simulink model "messageEvents_example1"  (R2024b)
settings: Solver=VariableStepAuto  StartTime=0.0  StopTime=10.0  RelTol=1e-3
undefined symbols (not defined in the file): Call, Function
settings Model: Creator=optimus  LastModifiedBy=optimus

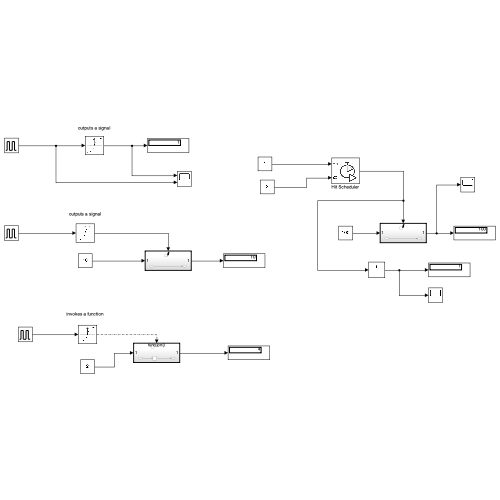
[thumbnail: Simulink's stored preview of the top-level diagram]
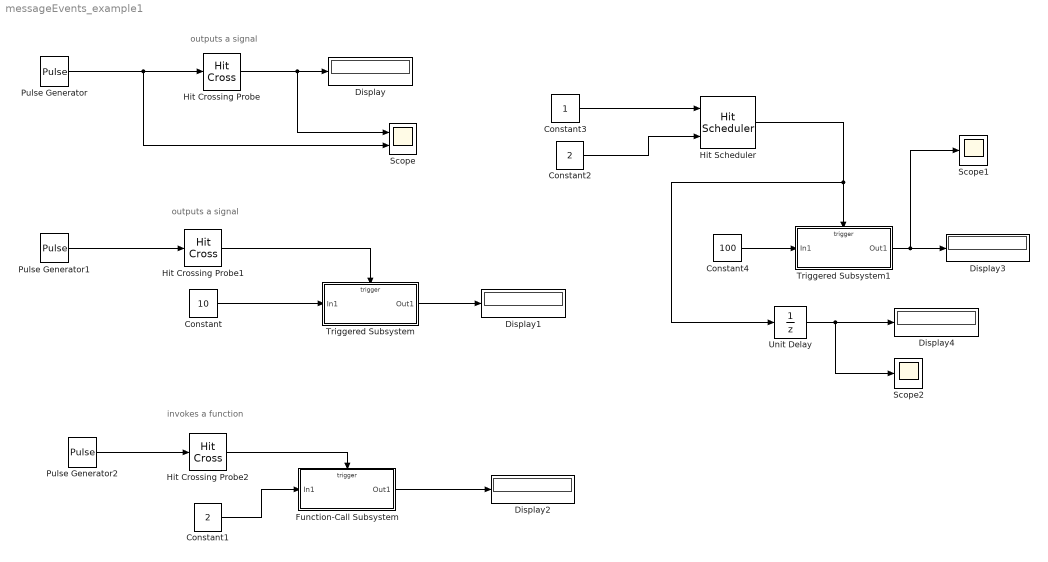
== system messageEvents_example1 ==
  note: invokes a function
  note: outputs a signal
  note: outputs a signal
  Constant : Constant  Value=10
  Constant1 : Constant  Value=2
  Constant2 : Constant  Value=2
  Constant3 : Constant  OutDataTypeStr=boolean
  Constant4 : Constant  Value=100
  Display{,1..4} (5 alike) : Display
  Function-Call Subsystem : Subsystem  TreatAsAtomicUnit=on
  Hit Crossing Probe : HitCross  HitCrossingDirection=rising
  Hit Crossing Probe1 : HitCross  HitCrossingDirection=rising
  Hit Crossing Probe2 : HitCross  HitCrossingDirection=rising  HitCrossingOutputType=Function-Call
  Hit Scheduler : HitScheduler
  Pulse Generator : DiscretePulseGenerator  PulseType=Time based  PulseWidth=50
  Pulse Generator1 : DiscretePulseGenerator  PulseType=Time based  PulseWidth=50
  Pulse Generator2 : DiscretePulseGenerator  PulseType=Time based  PulseWidth=50
  Scope : Scope  NumInputPorts=2
  Scope1 : Scope
  Scope2 : Scope
  Triggered Subsystem : Subsystem  TreatAsAtomicUnit=on
  Triggered Subsystem1 : Subsystem  TreatAsAtomicUnit=on
  Unit Delay : UnitDelay  SampleTime=-1  HasFrameUpgradeWarning=on
  wires:
  Pulse Generator/1 -> Scope/2, Hit Crossing Probe/1
  Hit Crossing Probe/1 -> Scope/1, Display/1
  Pulse Generator1/1 -> Hit Crossing Probe1/1
  Hit Crossing Probe1/1 -> Triggered Subsystem/Trigger
  Constant/1 -> Triggered Subsystem/1(In1)
  Triggered Subsystem/1(Out1) -> Display1/1
  Pulse Generator2/1 -> Hit Crossing Probe2/1
  Hit Crossing Probe2/1 -> Function-Call Subsystem/Trigger
  Constant1/1 -> Function-Call Subsystem/1(In1)
  Function-Call Subsystem/1(Out1) -> Display2/1
  Constant3/1 -> Hit Scheduler/1
  Constant2/1 -> Hit Scheduler/2
  Hit Scheduler/1 -> Unit Delay/1, Triggered Subsystem1/Trigger
  Constant4/1 -> Triggered Subsystem1/1(In1)
  Triggered Subsystem1/1(Out1) -> Scope1/1, Display3/1
  Unit Delay/1 -> Scope2/1, Display4/1

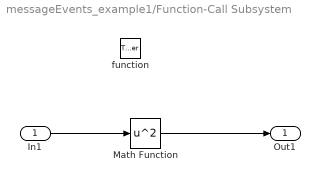
== system messageEvents_example1/Function-Call Subsystem ==
  In1 : Inport
  function : TriggerPort  TriggerType=function-call  VariantControl=(inherit)
  Math Function : Math  Operator=square
  Out1 : Outport
  wires:
  In1/1 -> Math Function/1
  Math Function/1 -> Out1/1

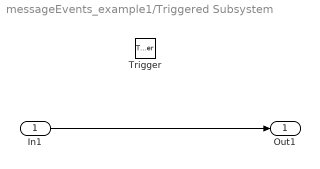
== system messageEvents_example1/Triggered Subsystem ==
  In1 : Inport
  Trigger : TriggerPort  VariantControl=(inherit)
  Out1 : Outport
  wires:
  In1/1 -> Out1/1

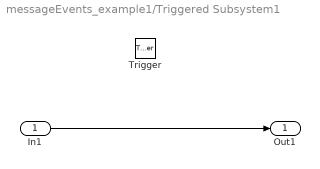
== system messageEvents_example1/Triggered Subsystem1 ==
  In1 : Inport
  Trigger : TriggerPort  VariantControl=(inherit)
  Out1 : Outport
  wires:
  In1/1 -> Out1/1
